simulink subsystem "StudentTemplateNew"  (R2025a)
settings: Solver=VariableStepAuto  StartTime=0.0  StopTime=10.0  RelTol=1e-3
libraries: eeGeneralControl x3
settings Model: Creator=JesseJabezArendse  LastModifiedBy=llamalulu

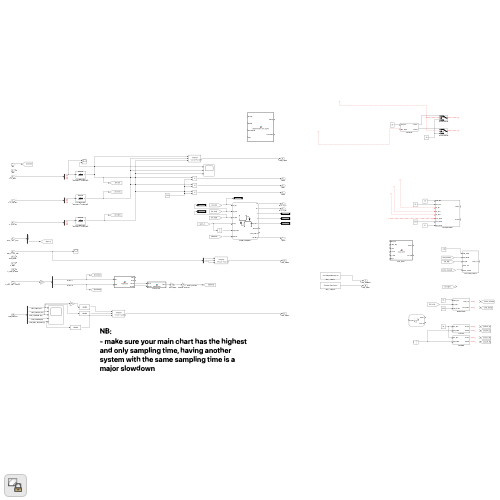
[thumbnail: Simulink's stored preview of the top-level diagram]
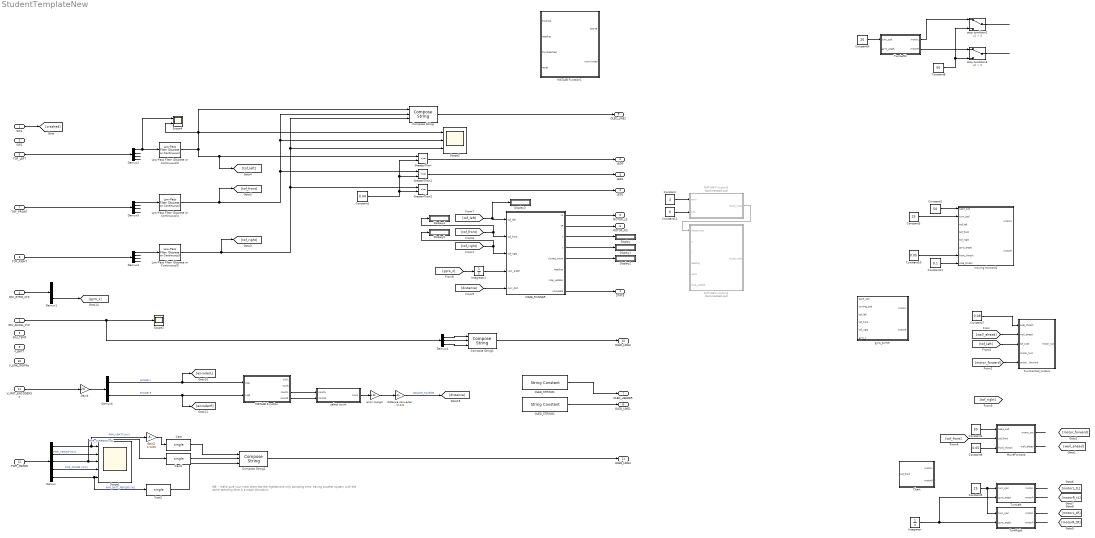
== system StudentTemplateNew ==
  note: NB:
      |
      | - make sure your main chart has the highest and only sampling time, having another system with the same sampling time is a major slowdown
  SW1 : Inport
  SW2 : Inport  Port=2
  IMU_ACCEL_XYZ : Inport  Port=3
  IMU_GYRO_XYZ : Inport  Port=4
  IMU_TEMP : Inport  Port=5
  TOF_LEFT : Inport  Port=6
  TOF_FRONT : Inport  Port=7
  TOF_RIGHT : Inport  Port=8
  V_BATT : Inport  Port=9
  V_LINE_DOWNs : Inport  Port=10
  V_MOT_ENCODERSs : Inport  Port=11
  PWR_METER : Inport  Port=12
  Cast : DataTypeConversion  OutDataTypeStr=single  SaturateOnIntegerOverflow=off  RndMeth=Floor
  Cast1 : DataTypeConversion  OutDataTypeStr=single  SaturateOnIntegerOverflow=off  RndMeth=Floor
  Cast2 : DataTypeConversion  OutDataTypeStr=single  SaturateOnIntegerOverflow=off  RndMeth=Floor
  Chart : Stateflow chart  TreatAsAtomicUnit=on
  Compose String : ComposeString  Format="\"L%1.2f F%1.2f R%1.2f\""
  Compose String1 : ComposeString  Format="\"X%2.1f  Y%2.1f  Z%2.1f\""
  Compose String2 : ComposeString  Format="\"%1.2fV  %3.0fmA  %2.0f%%\""
  Constant : Constant  Value=4
  Constant1 : Constant  Value=0.04  SampleTime=-1
  Constant10 : Constant  Value=0.05
  Constant11 : Constant  Value=0.1
  Constant12 : Constant  Value=6
  Constant2 : Constant  Value=50
  Constant3 : Constant  Value=25
  Constant4 : Constant  Value=50
  Constant5 : Constant  Value=25
  Constant6 : Constant  Value=0.05  SampleTime=-1
  Constant7 : Constant  Value=0.08  SampleTime=-1
  Constant8 : Constant  Value=50
  Constant9 : Constant  Value=20
  Demux : Demux  Outputs=5
  Demux1 : Demux  Outputs=3
  Demux2 : Demux
  Demux3 : Demux
  Demux4 : Demux  Outputs=3
  Demux5 : Demux
  Demux6 : Demux  Outputs=2
  Display{,1..5} (6 alike) : Display
  Gain2 : Gain  Gain=1/1000
  Gain4 : Gain  Gain=20
  GreaterThan : RelationalOperator  Operator=<=  OutDataTypeStr=boolean  RndMeth=Simplest  InputSameDT=off
  GreaterThan1 : RelationalOperator  Operator=<=  OutDataTypeStr=boolean  RndMeth=Simplest  InputSameDT=off
  GreaterThan2 : RelationalOperator  Operator=<=  OutDataTypeStr=boolean  RndMeth=Simplest  InputSameDT=off
  Integrator : Integrator
  Integrator1 : Integrator
  Low-Pass Filter (Discrete or Continuous)3 : eeGeneralControl/Low-Pass Filter (Discrete or Continuous)  K=1  T=0.1  B=inf  A=-inf  init_option=Inherited from block input  x0=0  Ts=-1
  Low-Pass Filter (Discrete or Continuous)4 : eeGeneralControl/Low-Pass Filter (Discrete or Continuous)  K=1  T=0.1  B=inf  A=-inf  init_option=Inherited from block input  x0=0  Ts=-1
  Low-Pass Filter (Discrete or Continuous)5 : eeGeneralControl/Low-Pass Filter (Discrete or Continuous)  K=1  T=0.1  B=inf  A=-inf  init_option=Inherited from block input  x0=0  Ts=-1
  MATLAB Function : MATLAB Function  TreatAsAtomicUnit=on  SystemSampleTime=0.01
  MATLAB Function1 : MATLAB Function  TreatAsAtomicUnit=on
  MATLAB Function2 : MATLAB Function  Commented=on  TreatAsAtomicUnit=on
  MATLAB Function3 : MATLAB Function  Commented=on  TreatAsAtomicUnit=on
  MAZE_RUNNER : Stateflow chart  TreatAsAtomicUnit=on
  MoveForward : Subsystem
  OLED_STRING1 : StringConstant  String="\"UCT MICROMOUSE '25\""
  OLED_STRING2 : StringConstant  String="\"Simulink Data Demo\""
  Scope1 : Scope  NumInputPorts=5
      settings: ActiveDisplayYMinimum=-437.5  ActiveDisplayYMaximum=3937.5  DataLoggingVariableName=ScopeData5
  Scope2 : Scope
      settings: DataLoggingVariableName=ScopeData6
  Scope3 : Scope  NumInputPorts=3
      settings: ActiveDisplayYMinimum=-0.018519426447002579  ActiveDisplayYMaximum=0.76884421439193007  DataLoggingVariableName=ScopeData3
  Scope4 : Scope  NumInputPorts=2
      settings: ActiveDisplayYMinimum=0.22759  ActiveDisplayYMaximum=0.52326  DataLoggingVariableName=ScopeData7
  TurnControl_motorL : Subsystem
  TurnLeft : Subsystem
  TurnLeft2 : Subsystem
  TurnRight : Subsystem
  distance converter : Gain  Gain=.214/8
  error margin : Gain  Gain=1.03
  "gyro_turner " : MATLAB Function  TreatAsAtomicUnit=on
  moving forward1 : Subsystem
  select count : MATLAB Function  TreatAsAtomicUnit=on
  stop condition2 : Switch  Criteria=u2 > Threshold  SaturateOnIntegerOverflow=off  InputSameDT=off
  stop condition3 : Switch  Criteria=u2 > Threshold  SaturateOnIntegerOverflow=off  InputSameDT=off
  STATE : Outport
  LED0 : Outport  Port=2
  LED1 : Outport  Port=3
  LED2 : Outport  Port=4
  MOTOR_LS : Outport  Port=5
  MOTOR_RS : Outport  Port=6
  OLED_HEADER : Outport  Port=7
  OLED_LINE1 : Outport  Port=8
  OLED_LINE2 : Outport  Port=9
  OLED_LINE3 : Outport  Port=10
  OLED_LINE4 : Outport  Port=11
  wires:
  OLED_STRING2/1 -> OLED_LINE1/1
  Compose String1/1 -> OLED_LINE3/1
  TOF_FRONT/1 -> Demux5/1
  GreaterThan1/1 -> LED1/1
  OLED_STRING1/1 -> OLED_HEADER/1
  Compose String/1 -> OLED_LINE2/1
  Constant1/1 -> GreaterThan2/2, GreaterThan1/2, GreaterThan/2
  GreaterThan2/1 -> LED2/1
  GreaterThan/1 -> LED0/1
  PWR_METER/1 -> Demux/1
  Demux/1 -> Scope1/1, Gain2/1  "PWR_VBATT [mV]"
  Demux/2 -> Scope1/2  "PWR_VSHUNT [mV]"
  Demux/3 -> Scope1/3, Cast1/1  "PWR_CURRENT [mA]"
  Demux/4 -> Scope1/4  "PWR_POWER [mW]"
  Demux/5 -> Scope1/5, Cast2/1  "PWR_BATT_PERCENT [%]"
  IMU_ACCEL_XYZ/1 -> Demux4/1, Scope2/1
  Demux4/1 -> Compose String1/1
  Demux4/2 -> Compose String1/2
  Demux4/3 -> Compose String1/3
  Compose String2/1 -> OLED_LINE4/1
  Gain2/1 -> Cast/1
  Cast/1 -> Compose String2/1
  Cast1/1 -> Compose String2/2
  Cast2/1 -> Compose String2/3
  TOF_RIGHT/1 -> Demux3/1
  TOF_LEFT/1 -> Demux2/1
  IMU_GYRO_XYZ/1 -> Demux1/1
  Demux1/3 -> [gyro_z]
  SW1/1 -> [crashed]
  Constant9/1 -> TurnLeft2/1(turn_spd)
  Constant8/1 -> stop condition2/3, stop condition3/3
  TurnLeft2/1(motorL) -> stop condition2/1
  stop condition3/1 -> ?
  TurnLeft2/2(motorR) -> stop condition3/1
  stop condition2/1 -> ?
  ? -> TurnLeft2/2(gyro_angle)
  ? -> stop condition3/2, stop condition2/2
  Constant11/1 -> moving forward1/8(side_thresh)
  Constant10/1 -> moving forward1/7(front_thresh)
  Constant3/1 -> moving forward1/2(turn_spd)
  Constant2/1 -> moving forward1/1(base_spd)
  ? -> moving forward1/6(gyro_angle)
  ? -> moving forward1/3(tof_left)
  ? -> moving forward1/5(tof_right)
  ? -> moving forward1/4(tof_front)
  Constant4/1 -> MoveForward/1(base_spd)
  Constant6/1 -> MoveForward/3(front_thresh)
  MoveForward/2(wall_ahead) -> ?
  Constant5/1 -> TurnLeft/1(turn_spd), TurnRight/1(turn_spd)
  Integrator/1 -> TurnRight/2(gyro_angle), TurnLeft/2(gyro_angle)
  [wall_ahead] -> TurnControl_motorL/2(wall_ahead)
  MoveForward/1(motor_out) -> ?
  [motor_forward] -> TurnControl_motorL/5(motor_forward)
  Constant7/1 -> TurnControl_motorL/1(side_thresh)
  [tof_front] -> MoveForward/2(tof_front)
  [tof_left] -> TurnControl_motorL/3(tof_side)
  TurnLeft/1(motorL) -> ?
  TurnLeft/2(motorR) -> ?
  TurnRight/2(motorR) -> ?
  TurnRight/1(motorL) -> ?
  Demux6/2 -> MATLAB Function/2(sigR), [encoderR]  "encoder R"
  Gain4/1 -> Demux6/1
  Demux6/1 -> MATLAB Function/1(sigL), [encoderL]  "encoder L"
  V_MOT_ENCODERSs/1 -> Gain4/1
  MAZE_RUNNER/2(vR) -> MOTOR_RS/1
  MAZE_RUNNER/1(vL) -> MOTOR_LS/1
  [tof_front] -> MAZE_RUNNER/2(tof_front), Display4/1
  [tof_right] -> MAZE_RUNNER/3(tof_right), Display5/1
  [tof_left] -> MAZE_RUNNER/1(tof_left), Display3/1
  [gyro_z] -> Integrator1/1
  Integrator1/1 -> MAZE_RUNNER/4(yaw_angle)
  select count/1(count) -> error margin/1
  error margin/1 -> distance converter/1
  MATLAB Function/3(countL) -> select count/1(countL)
  MATLAB Function/4(countR) -> select count/2(countR)
  [distance] -> MAZE_RUNNER/5(curr_dist)
  Demux2/4 -> ?
  Demux3/4 -> ?
  Demux2/1 -> Scope4/1, Low-Pass Filter (Discrete or Continuous)3/1
  Demux5/2 -> ?
  Demux2/2 -> ?
  Demux5/4 -> ?
  Demux3/3 -> ?
  Demux3/2 -> ?
  Demux5/3 -> ?
  Demux5/1 -> Low-Pass Filter (Discrete or Continuous)4/1
  Demux2/3 -> ?
  Demux3/1 -> Low-Pass Filter (Discrete or Continuous)5/1
  Low-Pass Filter (Discrete or Continuous)3/1 -> GreaterThan/1, [tof_left], Scope4/2, Compose String/1, Scope3/1
  Low-Pass Filter (Discrete or Continuous)4/1 -> GreaterThan1/1, Compose String/2, Scope3/2, [tof_front]
  Low-Pass Filter (Discrete or Continuous)5/1 -> GreaterThan2/1, Scope3/3, Compose String/3, [tof_right]
  MAZE_RUNNER/8(complete) -> STATE/1
  MAZE_RUNNER/3(x) -> Display/1
  MAZE_RUNNER/4(y) -> Display1/1
  MAZE_RUNNER/5(visited_count) -> Display2/1
  distance converter/1 -> [distance]  "distance_travelled"
  Constant/1 -> MATLAB Function3/1(rows)
  Constant12/1 -> MATLAB Function3/2(cols)
  MATLAB Function3/1(maze_map) -> MATLAB Function2/1("maze_map ")

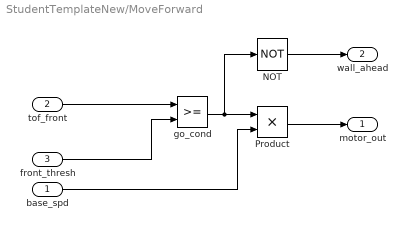
== system StudentTemplateNew/MoveForward ==
  base_spd : Inport
  tof_front : Inport  Port=2
  front_thresh : Inport  Port=3
  NOT : Logic  Operator=NOT  IconShape=distinctive  AllPortsSameDT=off  OutDataTypeStr=boolean
  Product : Product
  go_cond : RelationalOperator  OutDataTypeStr=boolean  RndMeth=Simplest  InputSameDT=off
  motor_out : Outport
  wall_ahead : Outport  Port=2
  wires:
  NOT/1 -> wall_ahead/1
  Product/1 -> motor_out/1
  base_spd/1 -> Product/2
  front_thresh/1 -> go_cond/2
  tof_front/1 -> go_cond/1
  go_cond/1 -> Product/1, NOT/1

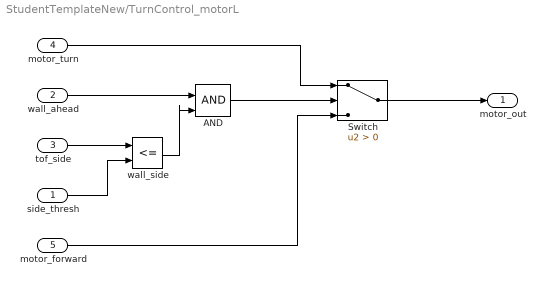
== system StudentTemplateNew/TurnControl_motorL ==
  side_thresh : Inport
  wall_ahead : Inport  Port=2
  tof_side : Inport  Port=3
  motor_turn : Inport  Port=4
  motor_forward : Inport  Port=5
  AND : Logic  IconShape=distinctive  AllPortsSameDT=off  OutDataTypeStr=boolean
  Switch : Switch  Criteria=u2 > Threshold  SaturateOnIntegerOverflow=off  InputSameDT=off
  wall_side : RelationalOperator  Operator=<=  OutDataTypeStr=boolean  RndMeth=Simplest  InputSameDT=off
  motor_out : Outport
  wires:
  wall_ahead/1 -> AND/1
  side_thresh/1 -> wall_side/2
  tof_side/1 -> wall_side/1
  Switch/1 -> motor_out/1
  AND/1 -> Switch/2
  wall_side/1 -> AND/2
  motor_turn/1 -> Switch/1
  motor_forward/1 -> Switch/3

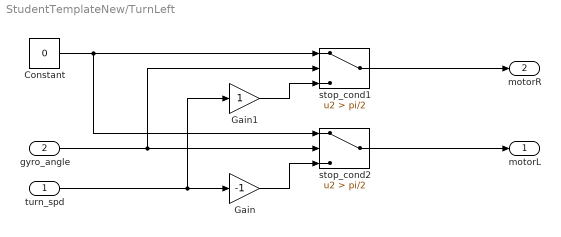
== system StudentTemplateNew/TurnLeft ==
  turn_spd : Inport
  gyro_angle : Inport  Port=2
  Constant : Constant  Value=0
  Gain : Gain  Gain=-1
  Gain1 : Gain
  stop_cond1 : Switch  Criteria=u2 > Threshold  Threshold=pi/2  SaturateOnIntegerOverflow=off  InputSameDT=off
  stop_cond2 : Switch  Criteria=u2 > Threshold  Threshold=pi/2  SaturateOnIntegerOverflow=off  InputSameDT=off
  motorL : Outport
  motorR : Outport  Port=2
  wires:
  gyro_angle/1 -> stop_cond2/2, stop_cond1/2
  stop_cond2/1 -> motorL/1
  Gain1/1 -> stop_cond1/3
  Gain/1 -> stop_cond2/3
  Constant/1 -> stop_cond2/1, stop_cond1/1
  stop_cond1/1 -> motorR/1
  turn_spd/1 -> Gain1/1, Gain/1

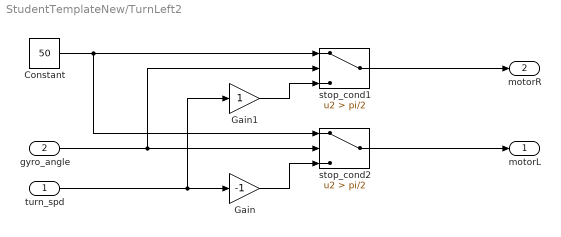
== system StudentTemplateNew/TurnLeft2 ==
  turn_spd : Inport
  gyro_angle : Inport  Port=2
  Constant : Constant  Value=50
  Gain : Gain  Gain=-1
  Gain1 : Gain
  stop_cond1 : Switch  Criteria=u2 > Threshold  Threshold=pi/2  SaturateOnIntegerOverflow=off  InputSameDT=off
  stop_cond2 : Switch  Criteria=u2 > Threshold  Threshold=pi/2  SaturateOnIntegerOverflow=off  InputSameDT=off
  motorL : Outport
  motorR : Outport  Port=2
  wires:
  gyro_angle/1 -> stop_cond2/2, stop_cond1/2
  stop_cond2/1 -> motorL/1
  Gain1/1 -> stop_cond1/3
  Gain/1 -> stop_cond2/3
  Constant/1 -> stop_cond2/1, stop_cond1/1
  stop_cond1/1 -> motorR/1
  turn_spd/1 -> Gain1/1, Gain/1

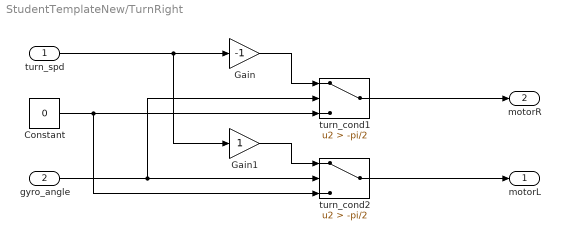
== system StudentTemplateNew/TurnRight ==
  turn_spd : Inport
  gyro_angle : Inport  Port=2
  Constant : Constant  Value=0
  Gain : Gain  Gain=-1
  Gain1 : Gain
  turn_cond1 : Switch  Criteria=u2 > Threshold  Threshold=-pi/2  SaturateOnIntegerOverflow=off  InputSameDT=off
  turn_cond2 : Switch  Criteria=u2 > Threshold  Threshold=-pi/2  SaturateOnIntegerOverflow=off  InputSameDT=off
  motorL : Outport
  motorR : Outport  Port=2
  wires:
  turn_spd/1 -> Gain/1, Gain1/1
  turn_cond1/1 -> motorR/1
  Constant/1 -> turn_cond2/3, turn_cond1/3
  Gain1/1 -> turn_cond2/1
  Gain/1 -> turn_cond1/1
  turn_cond2/1 -> motorL/1
  gyro_angle/1 -> turn_cond1/2, turn_cond2/2

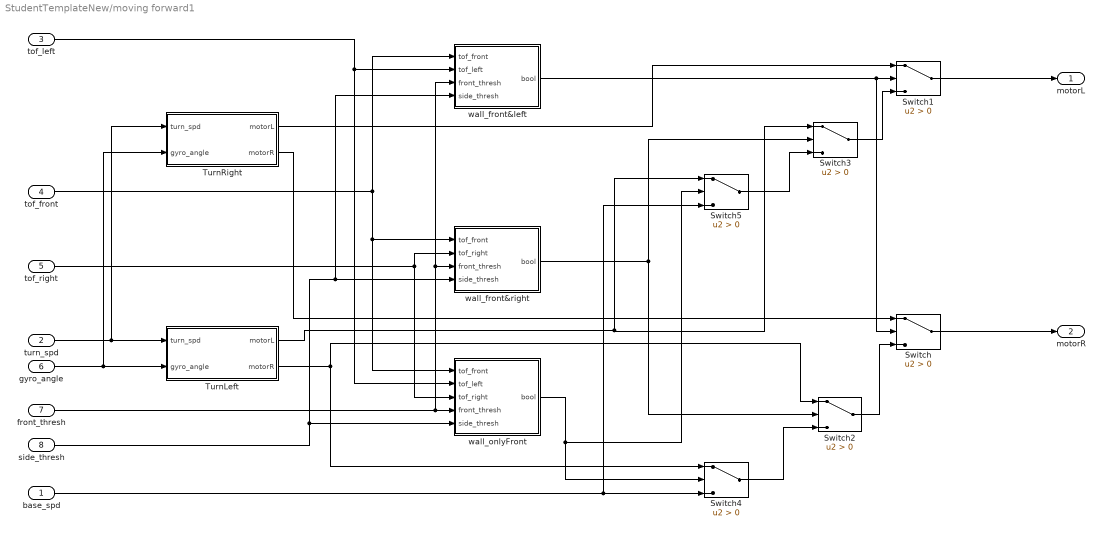
== system StudentTemplateNew/moving forward1 ==
  base_spd : Inport
  turn_spd : Inport  Port=2
  tof_left : Inport  Port=3
  tof_front : Inport  Port=4
  tof_right : Inport  Port=5
  gyro_angle : Inport  Port=6
  front_thresh : Inport  Port=7
  side_thresh : Inport  Port=8
  Switch{,1..5} (6 alike) : Switch  Criteria=u2 > Threshold  SaturateOnIntegerOverflow=off  InputSameDT=off
  TurnLeft : Subsystem
  TurnRight : Subsystem
  wall_front&left : Subsystem
  wall_front&right : Subsystem
  wall_onlyFront : Subsystem
  motorL : Outport
  motorR : Outport  Port=2
  wires:
  tof_left/1 -> wall_onlyFront/2(tof_left), wall_front&left/2(tof_left)
  Switch/1 -> motorR/1
  Switch5/1 -> Switch3/3
  Switch2/1 -> Switch/3
  Switch1/1 -> motorL/1
  TurnRight/1(motorL) -> Switch1/1
  wall_front&right/1(bool) -> Switch3/2, Switch2/2
  Switch3/1 -> Switch1/3
  TurnLeft/1(motorL) -> Switch3/1, Switch5/1
  gyro_angle/1 -> TurnRight/2(gyro_angle), TurnLeft/2(gyro_angle)
  TurnLeft/2(motorR) -> Switch2/1, Switch4/1
  turn_spd/1 -> TurnRight/1(turn_spd), TurnLeft/1(turn_spd)
  tof_front/1 -> wall_front&left/1(tof_front), wall_onlyFront/1(tof_front), wall_front&right/1(tof_front)
  Switch4/1 -> Switch2/3
  wall_onlyFront/1(bool) -> Switch5/2, Switch4/2
  TurnRight/2(motorR) -> Switch/1
  base_spd/1 -> Switch5/3, Switch4/3
  tof_right/1 -> wall_onlyFront/3(tof_right), wall_front&right/2(tof_right)
  wall_front&left/1(bool) -> Switch/2, Switch1/2
  side_thresh/1 -> wall_front&left/4(side_thresh), wall_front&right/4(side_thresh), wall_onlyFront/5(side_thresh)
  front_thresh/1 -> wall_front&left/3(front_thresh), wall_front&right/3(front_thresh), wall_onlyFront/4(front_thresh)

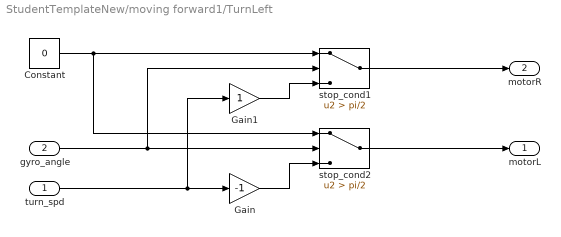
== system StudentTemplateNew/moving forward1/TurnLeft ==
  turn_spd : Inport
  gyro_angle : Inport  Port=2
  Constant : Constant  Value=0
  Gain : Gain  Gain=-1
  Gain1 : Gain
  stop_cond1 : Switch  Criteria=u2 > Threshold  Threshold=pi/2  SaturateOnIntegerOverflow=off  InputSameDT=off
  stop_cond2 : Switch  Criteria=u2 > Threshold  Threshold=pi/2  SaturateOnIntegerOverflow=off  InputSameDT=off
  motorL : Outport
  motorR : Outport  Port=2
  wires:
  gyro_angle/1 -> stop_cond2/2, stop_cond1/2
  stop_cond2/1 -> motorL/1
  Gain1/1 -> stop_cond1/3
  Gain/1 -> stop_cond2/3
  Constant/1 -> stop_cond2/1, stop_cond1/1
  stop_cond1/1 -> motorR/1
  turn_spd/1 -> Gain1/1, Gain/1

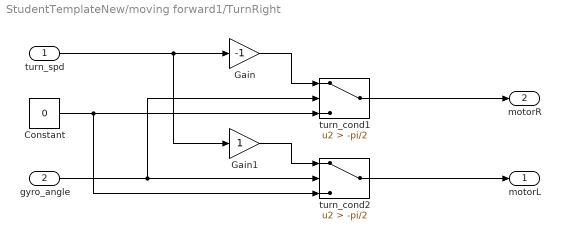
== system StudentTemplateNew/moving forward1/TurnRight ==
  turn_spd : Inport
  gyro_angle : Inport  Port=2
  Constant : Constant  Value=0
  Gain : Gain  Gain=-1
  Gain1 : Gain
  turn_cond1 : Switch  Criteria=u2 > Threshold  Threshold=-pi/2  SaturateOnIntegerOverflow=off  InputSameDT=off
  turn_cond2 : Switch  Criteria=u2 > Threshold  Threshold=-pi/2  SaturateOnIntegerOverflow=off  InputSameDT=off
  motorL : Outport
  motorR : Outport  Port=2
  wires:
  gyro_angle/1 -> turn_cond2/2, turn_cond1/2
  turn_cond2/1 -> motorL/1
  Gain/1 -> turn_cond1/1
  Gain1/1 -> turn_cond2/1
  Constant/1 -> turn_cond1/3, turn_cond2/3
  turn_cond1/1 -> motorR/1
  turn_spd/1 -> Gain1/1, Gain/1

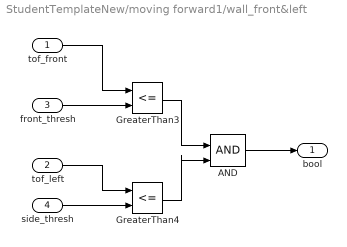
== system StudentTemplateNew/moving forward1/wall_front&left ==
  tof_front : Inport
  tof_left : Inport  Port=2
  front_thresh : Inport  Port=3
  side_thresh : Inport  Port=4
  AND : Logic  IconShape=distinctive  AllPortsSameDT=off  OutDataTypeStr=boolean
  GreaterThan3 : RelationalOperator  Operator=<=  OutDataTypeStr=boolean  RndMeth=Simplest  InputSameDT=off
  GreaterThan4 : RelationalOperator  Operator=<=  OutDataTypeStr=boolean  RndMeth=Simplest  InputSameDT=off
  bool : Outport
  wires:
  AND/1 -> bool/1
  tof_front/1 -> GreaterThan3/1
  side_thresh/1 -> GreaterThan4/2
  GreaterThan3/1 -> AND/1
  front_thresh/1 -> GreaterThan3/2
  tof_left/1 -> GreaterThan4/1
  GreaterThan4/1 -> AND/2

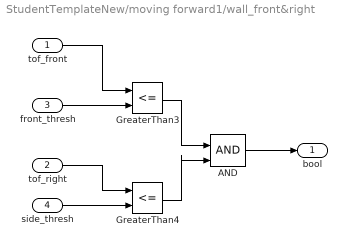
== system StudentTemplateNew/moving forward1/wall_front&right ==
  tof_front : Inport
  tof_right : Inport  Port=2
  front_thresh : Inport  Port=3
  side_thresh : Inport  Port=4
  AND : Logic  IconShape=distinctive  AllPortsSameDT=off  OutDataTypeStr=boolean
  GreaterThan3 : RelationalOperator  Operator=<=  OutDataTypeStr=boolean  RndMeth=Simplest  InputSameDT=off
  GreaterThan4 : RelationalOperator  Operator=<=  OutDataTypeStr=boolean  RndMeth=Simplest  InputSameDT=off
  bool : Outport
  wires:
  AND/1 -> bool/1
  tof_front/1 -> GreaterThan3/1
  side_thresh/1 -> GreaterThan4/2
  GreaterThan3/1 -> AND/1
  front_thresh/1 -> GreaterThan3/2
  tof_right/1 -> GreaterThan4/1
  GreaterThan4/1 -> AND/2

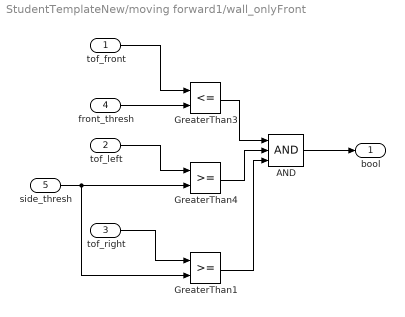
== system StudentTemplateNew/moving forward1/wall_onlyFront ==
  tof_front : Inport
  tof_left : Inport  Port=2
  tof_right : Inport  Port=3
  front_thresh : Inport  Port=4
  side_thresh : Inport  Port=5
  AND : Logic  Inputs=3  IconShape=distinctive  AllPortsSameDT=off  OutDataTypeStr=boolean
  GreaterThan1 : RelationalOperator  OutDataTypeStr=boolean  RndMeth=Simplest  InputSameDT=off
  GreaterThan3 : RelationalOperator  Operator=<=  OutDataTypeStr=boolean  RndMeth=Simplest  InputSameDT=off
  GreaterThan4 : RelationalOperator  OutDataTypeStr=boolean  RndMeth=Simplest  InputSameDT=off
  bool : Outport
  wires:
  AND/1 -> bool/1
  tof_front/1 -> GreaterThan3/1
  GreaterThan3/1 -> AND/1
  front_thresh/1 -> GreaterThan3/2
  tof_left/1 -> GreaterThan4/1
  GreaterThan4/1 -> AND/2
  tof_right/1 -> GreaterThan1/1
  side_thresh/1 -> GreaterThan1/2, GreaterThan4/2
  GreaterThan1/1 -> AND/3

== stateflow chart StudentTemplateNew/MAZE_RUNNER ==
  state INIT
    entry:
    vL = 0;
    vR = 0;
    x = 0; y = 0;
    heading = 1; % EAST
    visited_count = 1;
    yaw_tol = 0.1; % radians (~6°)
    all_paths_visited = false;
    just_turned = false;
  state SCAN_ENV
    entry:
    left_open  = (tof_left  > wall_threshold);
    front_open = (tof_front > wall_threshold);
    right_open = (tof_right > wall_threshold);
    during:
    vL = 0;
    vR = 0;
    map_update = true;
  state CHECK_DONE
    entry:
    if visited_count >= TOTAL_CELLS
    all_paths_visited = true;
    next_state = NextState.END;
    else
    next_state = NextState.SCAN_ENV;
    end
  state END
    vL = 0;
    vR = 0;
    complete = true;
    %blink_LED(SUCCESS);
  state DECIDE
    entry:
    %left_open = false;
    %front_open = false;
    %right_open = false;
    if left_open
    next_state = NextState.TURN_LEFT;
    elseif front_open
    next_state = NextState.MOVE_FORWARD;
    elseif right_open
    next_state = NextState.TURN_RIGHT;
    else
    next_state = NextState.TURN_BACK;
    end
  state TURN_LEFT
    entry:
    start_yaw = yaw_angle;          % record entry angle
    target_delta = pi/2;            % 90° turn
    vL = -TURN_SPEED;
    vR = TURN_SPEED;
    during:
    delta_yaw = wrapToPi(yaw_angle - start_yaw);  % normalize to [-π, π]
    if abs(delta_yaw) >= target_delta
    heading = mod(heading + 3, 4);
    vL = 0;
    vR = 0;
    just_turned = true;
    next_state = NextState.MOVE_FORWARD;
    end
  state TURN_RIGHT
    entry:
    start_yaw = yaw_angle;          % record entry angle
    target_delta = pi/2;            % 90° turn
    vL = TURN_SPEED;
    vR = -TURN_SPEED;
    during:
    delta_yaw = wrapToPi(start_yaw - yaw_angle);  % normalize to [-π, π]
    if abs(delta_yaw) >= target_delta
    heading = mod(heading + 1, 4);
    vL = 0;
    vR = 0;
    just_turned = true;
    next_state = NextState.MOVE_FORWARD;
    end
  state TURN_BACK
    entry:
    start_yaw = yaw_angle;          % record entry angle
    target_delta = pi;            % 180° turn
    vL = -TURN_SPEED;
    vR = TURN_SPEED;
    during:
    delta_yaw = yaw_angle - start_yaw;  % normalize to [-π, π]
    if abs(delta_yaw) >= target_delta
    heading = mod(heading + 2, 4);
    vL = 0;
    vR = 0;
    just_turned = true;
    next_state = NextState.MOVE_FORWARD;
    end
  state MOVE_FORWARD
    entry:
    start_dist = curr_dist;           % starting distance (m)
    last_left_open  = left_open;
    last_right_open = right_open;
    side_open_event = false;
    vL = BASE_SPEED;
    vR = BASE_SPEED;
    during:
    left_open  = (tof_left  > wall_threshold);
    right_open = (tof_right > wall_threshold);
    dist_travelled = curr_dist - start_dist;
    % --- Detect side wall opened (blocked -> open) ---
    if ((left_open && ~last_left_open) || (right_open && ~last_right_open)) && just_turned == false
    start_dist = curr_dist;          % new reference
    side_open_event = true;          % remember that we saw an opening
    end
    % Always update last states
    last_left_open  = left_open;
    last_right_open = right_open;
    % --- Stop conditions ---
    if side_open_event && (curr_dist - start_dist) >= 0.16
    % 0.16 m after a new opening
    vL = 0; vR = 0;
    side_open_event = false;     % reset flag
    cond = 1;
    just_turned = false;
    next_state = NextState.UPDATE_POSITION;
    elseif tof_front <= 0.04
    % Front wall very close
    vL = 0; vR = 0;
    cond = 2;
    just_turned = false;
    next_state = NextState.UPDATE_POSITION;
    elseif (curr_dist - start_dist) >= (cell_length + 0.023)
    % Normal full-cell traversal
    vL = 0; vR = 0;
    cond = 3;
    just_turned = false;
    next_state = NextState.UPDATE_POSITION;
    end
  state UPDATE_POSITION
    entry:
    switch heading
    case 0
    y = y + 1; % NORTH
    case 1
    x = x + 1; % EAST
    case 2
    y = y - 1; % SOUTH
    case 3
    x = x - 1; % WEST
    end
    visited_count = visited_count + 1;
    map_update = true;
    next_state = NextState.CHECK_DONE;
  (default) -> INIT
  CHECK_DONE -> END [order 1] : [next_state == NextState.END]
  INIT -> SCAN_ENV : after(1, sec)
  CHECK_DONE -> SCAN_ENV [order 2] : [next_state == NextState.SCAN_ENV]
  UPDATE_POSITION -> CHECK_DONE : [next_state == NextState.CHECK_DONE]
  SCAN_ENV -> DECIDE
  DECIDE -> TURN_LEFT [order 4] : [next_state == NextState.TURN_LEFT]
  DECIDE -> TURN_BACK [order 3] : [next_state == NextState.TURN_BACK]
  DECIDE -> MOVE_FORWARD [order 1] : [next_state == NextState.MOVE_FORWARD]
  DECIDE -> TURN_RIGHT [order 2] : [next_state == NextState.TURN_RIGHT]
  TURN_RIGHT -> MOVE_FORWARD : [next_state == NextState.MOVE_FORWARD]
  TURN_LEFT -> MOVE_FORWARD : [next_state == NextState.MOVE_FORWARD]
  TURN_BACK -> MOVE_FORWARD : [next_state == NextState.MOVE_FORWARD]
  MOVE_FORWARD -> UPDATE_POSITION : [next_state == NextState.UPDATE_POSITION]
  data: tof_left input double; tof_front input double; tof_right input double; yaw_angle input; vL output; vR output; x output; y output; visited_count output double; heading output; map_update output boolean; complete output boolean; start_dist local; cell_length constant double =0.2; yaw_tol local; wall_threshold constant double =0.12; left_open local boolean; right_open local boolean; front_open local boolean; all_paths_visited local boolean; curr_dist input; TURN_SPEED constant double =60; TOTAL_CELLS constant double =24; BASE_SPEED constant double =80; next_state local Enum: NextState =NextState.NONE; start_yaw local; target_delta local; delta_yaw local; last_left_open local; last_right_open local; dist_travelled local; cond local; side_open_event local; just_turned local
  data tof_left settings: description=ToF sensor distances (m)
  data tof_front settings: description=ToF sensor distances (m)
  data tof_right settings: description=ToF sensor distances (m)
  data yaw_angle settings: description=Integrated yaw
  data vL settings: description=Left and right motor speeds
  data vR settings: description=Left and right motor speeds
  data x settings: description=Current cell coordinates
  data y settings: description=Current cell coordinates
  data visited_count settings: description=Number of visited cells
  data heading settings: description=Discrete heading (0=N,1=E,2=S,3=W)
  data start_dist settings: description=Encoder baseline before move
  data cell_length settings: description=~8 ticks (distance for one cell)
  data yaw_tol settings: description=Angle tolerance (e.g., 0.1 rad)
  data wall_threshold settings: description=Distance threshold for wall detection
  function ?:
    | function

== matlab function StudentTemplateNew/select count ==
  data: countL input; count output; countR input
function count = selectCount(countL, countR)
% countL, countR : encoder tick counts
% count          : best encoder count

% Force doubles (avoid fi issues)
countL = double(countL);
countR = double(countR);

% Default
count = 0;

% Fault-tolerant distance estimate
if max(countL, countR) == 0
    % Avoid division by zero on startup
    count = 0;
elseif abs(countL - countR) < 0.5 * max(countL, countR)
    % If both encoders agree within 50%, take average
    count = (countL + countR)/2;
else
    % If one encoder lags badly, trust the larger one
    count = max(countL, countR);
end

== matlab function StudentTemplateNew/MATLAB Function1 ==
  data: frontToF input; STATE output; heading input; TurnReached input; reset input; numVisited output
function [STATE, numVisited] = MazeTracker_ToF_signed(frontToF, heading, TurnReached, reset)
%#codegen
% ToF-based maze tracker for 4x6 maze
% Tracks visited blocks accurately, handles multiple consecutive turns
% Inputs:
%   frontToF    - distance to front wall (m)
%   heading     - current heading (rad)
%   TurnReached - 1 if turning, 0 otherwise
%   reset       - 1 to reset maze map
% Outputs:
%   STATE       - 1 if all blocks visited, 0 otherwise
%   numVisited  - total number of blocks visited

maze_rows = 4;
maze_cols = 6;
block_size = 0.2;

persistent row col visited_map prevFront prevTurn accumX accumY
if isempty(row) || reset
    row = 1; col = 1;                       % bottom-left
    visited_map = zeros(maze_rows, maze_cols);
    visited_map(row, col) = 1;
    prevFront = frontToF;
    prevTurn = 0;
    accumX = block_size/2;                  % start halfway in first block
    accumY = block_size/2;
end

% detect turn start/stop
turnStarted = (~prevTurn && TurnReached);
prevTurn = TurnReached;

% accumulate movement only when not turning, or just started a turn
if ~TurnReached || turnStarted
    delta = prevFront - frontToF;

    % signed X/Y movement based on heading
    deltaX = delta * cos(heading);
    deltaY = delta * sin(heading);

    accumX = accumX + deltaX;
    accumY = accumY + deltaY;
end
prevFront = frontToF;

% compute number of blocks crossed along each axis
colsCrossed = floor(accumX / block_size);
rowsCrossed = floor(accumY / block_size);

% update col/row with sign
if colsCrossed ~= 0
    col = min(max(col + sign(accumX) * abs(colsCrossed), 1), maze_cols);
end
if rowsCrossed ~= 0
    row = min(max(row + sign(accumY) * abs(rowsCrossed), 1), maze_rows);
end

% mark new block as visited
visited_map(row, col) = 1;

% subtract counted blocks from accumulators
accumX = accumX - colsCrossed * block_size;
accumY = accumY - rowsCrossed * block_size;

% outputs
numVisited = sum(visited_map(:));
STATE = double(numVisited == maze_rows * maze_cols);

end

== matlab function StudentTemplateNew/MATLAB Function2 ==
  data: maze_map input; maze_map output; x input; y input; heading input; walls input; map_update input

function maze_map = updateMazeMap(maze_map, x, y, heading, walls, map_update)
    % updateMazeMap - Updates maze map data for micromouse navigation
    %
    % Inputs:
    %   maze_map   - Structure array storing maze data (initialize with initMazeMap)
    %   x          - Current x coordinate of mouse
    %   y          - Current y coordinate of mouse
    %   heading    - Current heading of mouse (0=N, 90=E, 180=S, 270=W)
    %   walls      - Structure with fields: N, S, E, W (1=wall, 0=no wall)
    %   map_update - Boolean flag to trigger update
    %
    % Output:
    %   maze_map   - Updated maze map structure
    
    % Only update if map_update is true
    if ~map_update
        return;
    end
    
    % Validate coordinates are within bounds
    if x < 1 || x > size(maze_map, 2) || y < 1 || y > size(maze_map, 1)
        warning('Coordinates (%d, %d) out of bounds', x, y);
        return;
    end
    
    % Update the cell data
    maze_map(y, x).x = x;
    maze_map(y, x).y = y;
    maze_map(y, x).heading = heading;
    maze_map(y, x).walls.N = walls.N;
    maze_map(y, x).walls.S = walls.S;
    maze_map(y, x).walls.E = walls.E;
    maze_map(y, x).walls.W = walls.W;
    maze_map(y, x).visited = true;
end

== matlab function StudentTemplateNew/MATLAB Function3 ==
  data: rows input; maze_map output Bus: <object name> [..100]; cols input
function maze_map = initMazeMap(rows, cols)
    % initMazeMap - Initialize empty maze map structure
    %
    % Inputs:
    %   rows - Number of rows in maze
    %   cols - Number of columns in maze
    %
    % Output:
    %   maze_map - Initialized maze map structure array
    
    % Create empty structure for one cell
    cell_template = struct('x', 0, 'y', 0, 'heading', 0, ...
                          'walls', struct('N', 0, 'S', 0, 'E', 0, 'W', 0), ...
                          'visited', false);
    
    % Create array of structures
    maze_map = repmat(cell_template, rows, cols);
    
    % Initialize coordinates for each cell
    for i = 1:rows
        for j = 1:cols
            maze_map(i, j).x = j;
            maze_map(i, j).y = i;
        end
    end
end

== matlab function StudentTemplateNew/gyro_turner  ==
  settings: updateMethod=DISCRETE
  data: motorL output; motorR output; base_spd input; turning_spd input; tof_left input; tof_front input; tof_right input; gyro_z input
function [motorL, motorR] = maze_drive(base_spd, turning_spd, tof_left, tof_front, tof_right, gyro_z)
%#codegen

% Thresholds
front_thresh = 0.08; 
side_thresh  = 0.1;  

% Persistent state for turns
persistent turning turn_dir target_angle
if isempty(turning)
    turning = false;
    turn_dir = 0;       % 1 = left, -1 = right
    target_angle = 0;
end

% Default motors (stop if no rule matches)
motorL = 0;
motorR = 0;

if turning
    % --- Currently in a turn ---
    if turn_dir == 1
        % Left turn (CCW)
        if gyro_z < target_angle
            motorL =  -turning_spd;
            motorR = turning_spd;
        else
            turning = false; % Done turning
        end
    elseif turn_dir == -1
        % Right turn (CW)
        if gyro_z > target_angle
            motorL = turning_spd;
            motorR = -turning_spd;
        else
            turning = false; % Done turning
        end
    end

else
    % --- Not currently turning, decide what to do ---
    if tof_front < front_thresh
        % Wall ahead
        if (tof_left < side_thresh && tof_right < side_thresh)
            % Dead end -> reverse
            motorL = -base_spd;
            motorR = -base_spd;
        elseif (tof_left < side_thresh && tof_right > side_thresh)
            % Prefer right turn
            turning     = true;
            turn_dir    = -1;
            target_angle = gyro_z - pi/2;
        elseif (tof_left > side_thresh && tof_right < side_thresh)
            % Prefer left turn
            turning     = true;
            turn_dir    = 1;
            target_angle = gyro_z + pi/2;
        else
            % If both sides open -> prioritise left
            turning     = true;
            turn_dir    = 1;
            target_angle = gyro_z + pi/2;
        end
    else
        % Path clear -> go forward
        motorL = base_spd;
        motorR = base_spd;
    end
end
end

== matlab function StudentTemplateNew/MATLAB Function ==
  data: sigL input; tickL output; sigR input; tickR output; countL output; countR output
function [tickL, tickR, countL, countR] = myEncoder(sigL, sigR)
% sigL, sigR : latest ADC values
% tickL, tickR : 1 when tick detected, else 0
% countL, countR : running tick counts

% Force doubles
sigL = double(sigL);
sigR = double(sigR);

% PARAMETERS
N = 7;                   % window length
debounce_samples = 10;   % ~10 samples = 10 ms at 1 kHz
offset = 0.005;            % fixed offset above running average

% Persistent state
persistent bufL bufR idx countL_int countR_int debL debR init
if isempty(init)
    bufL = sigL*ones(N,1,'double');
    bufR = sigR*ones(N,1,'double');
    idx = 1;
    countL_int = 0; countR_int = 0;
    debL = 0; debR = 0;
    init = true;
end

% Insert new values into circular buffers
bufL(idx) = sigL;
bufR(idx) = sigR;
idx = idx + 1;
if idx > N, idx = 1; end

% Compute running averages
avgL = mean(bufL);
avgR = mean(bufR);

% Init outputs
tickL = false;
tickR = false;

% --- Left detection ---
if debL > 0
    debL = debL - 1;
else
    if sigL > avgL + offset
        tickL = true;
        countL_int = countL_int + 1;
        debL = debounce_samples;
    end
end

% --- Right detection ---
if debR > 0
    debR = debR - 1;
else
    if sigR > avgR + offset
        tickR = true;
        countR_int = countR_int + 1;
        debR = debounce_samples;
    end
end

% Outputs
countL = countL_int;
countR = countR_int;

== stateflow chart StudentTemplateNew/Chart ==
  state Stop
    entry:
    motorL=0;
    motorR=0;
  state MoveForward
    entry:
    motorL=50;
    motorR=50;
  state TurnLeft
    entry:
    motorL=-25;
    motorR=25;
  state TurnRight
    entry:
    motorL=25;
    motorR=-25;
  state Reverse
    entry:
    motorL=-50;
    motorR=-50;
  (default) -> MoveForward
  data: turning_spd local =25; tof_front input; motorL output; motorR output
